simulink model "quadcop_flat"  (R2025b)
settings: Solver=ode4  StartTime=0.0  StopTime=40  FixedStep=Ts_inner  RelTol=1e-3
InitFcn:
  | fctrl = init_flatness(quadcop);
  | [mahony, luen] = init_estimator(fctrl.Ts_slow); % Ts_slow = 0.01 = Ts_gcs
  | xi0 = [quadcop.x0; quadcop.v0]; % Luenberger-Startzustand [p;v]
  | link_flat_params = init_link_flat(quadcop, Ts_inner);
undefined symbols (not defined in the file): quadcop, Ts_gcs, Ts_inner
settings Model: DataDictionary=project.sldd  Creator=Rakete  LastModifiedBy=Rakete

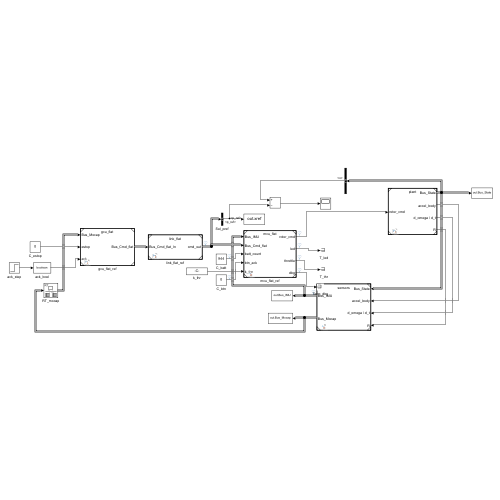
[thumbnail: Simulink's stored preview of the top-level diagram]
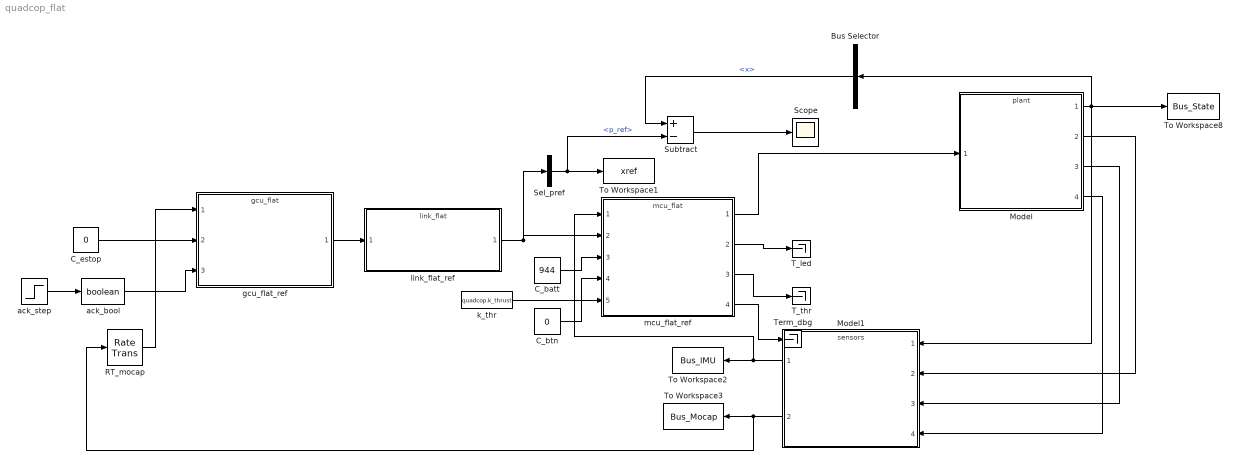
== system quadcop_flat ==
  Bus Selector : BusSelector  OutputSignals=x
  C_batt : Constant  Value=944
  C_btn : Constant  Value=0  OutDataTypeStr=boolean
  C_estop : Constant  Value=0  OutDataTypeStr=uint8
  Model : ModelReference  ModelNameDialog=plant.slx  SimulationMode=Normal  ModelReferenceVersion=1.211
  Model1 : ModelReference  ModelNameDialog=sensors.slx  SimulationMode=Normal  ModelReferenceVersion=1.89
  RT_mocap : RateTransition  OutPortSampleTime=Ts_gcs
  Scope : Scope
      settings: ActiveDisplayYMinimum=-0.18860034487092139  ActiveDisplayYMaximum=0.19828382929873062  DataLoggingVariableName=scope_sig
  Sel_pref : BusSelector  OutputSignals=p_ref
  Subtract : Sum  Inputs=+-
  T_led : Terminator
  T_thr : Terminator
  Term_dbg : Terminator
  To Workspace1 : ToWorkspace  VariableName=xref  SaveFormat=Timeseries  SampleTime=Ts_gcs
  To Workspace2 : ToWorkspace  VariableName=Bus_IMU  SaveFormat=Timeseries  SampleTime=Ts_gcs
  To Workspace3 : ToWorkspace  VariableName=Bus_Mocap  SaveFormat=Timeseries  SampleTime=Ts_gcs
  To Workspace8 : ToWorkspace  VariableName=Bus_State  SaveFormat=Timeseries  SampleTime=fctrl.Ts_slow
  ack_bool : DataTypeConversion  OutDataTypeStr=boolean  SaturateOnIntegerOverflow=off  RndMeth=Floor
  ack_step : Step  Description=Quittierung bei t = 1 s: steigende ack-Flanke schaltet die MCU scharf (bootet gekillt).  SampleTime=Ts_gcs
  gcu_flat_ref : ModelReference  ModelNameDialog=gcu_flat  ParameterArgumentNames=drone_idx  UsingDefaultArgumentValue=0  SimulationMode=Normal  ModelReferenceVersion=1.330
  k_thr : Constant  Value=quadcop.k_thrust  OutDataTypeStr=double  SampleTime=Ts_inner
  link_flat_ref : ModelReference  ModelNameDialog=link_flat  SimulationMode=Normal  ModelReferenceVersion=1.139
  mcu_flat_ref : ModelReference  ModelNameDialog=mcu_flat  SimulationMode=Normal  ModelReferenceVersion=1.333
  wires:
  link_flat_ref/1 -> mcu_flat_ref/2, Sel_pref/1
  C_estop/1 -> gcu_flat_ref/2
  gcu_flat_ref/1 -> link_flat_ref/1
  RT_mocap/1 -> gcu_flat_ref/1
  Sel_pref/1 -> Subtract/2, To Workspace1/1  "<p_ref>"
  C_batt/1 -> mcu_flat_ref/3
  Model/3 -> Model1/3
  Model1/2 -> RT_mocap/1, To Workspace3/1
  C_btn/1 -> mcu_flat_ref/4
  Subtract/1 -> Scope/1
  mcu_flat_ref/2 -> T_led/1
  mcu_flat_ref/1 -> Model/1
  mcu_flat_ref/3 -> T_thr/1
  Bus Selector/1 -> Subtract/1  "<x>"
  Model/2 -> Model1/2
  Model1/1 -> mcu_flat_ref/1, To Workspace2/1
  Model/1 -> To Workspace8/1, Model1/1, Bus Selector/1
  Model/4 -> Model1/4
  mcu_flat_ref/4 -> Term_dbg/1
  ack_step/1 -> ack_bool/1
  ack_bool/1 -> gcu_flat_ref/3
  k_thr/1 -> mcu_flat_ref/5
